simulink model "AT_and_specifications_artificial"  (R2019b)
settings: Solver=FixedStepAuto  StartTime=0.0  StopTime=10.0  FixedStep=fixedStepSize  RelTol=1e-3
settings Model: Creator=JEDDELAN  LastModifiedBy=jeddelan
settings DataIOCC: ReturnWorkspaceOutputs=off
settings DebuggingCC: ArithmeticOperatorsInVariantConditions=warning
settings SFSimCC: SimUseLocalCustomCode=off  CustomCodeUndefinedFunction=UseInterfaceOnly
settings RTWCC: RTWUseLocalCustomCode=off

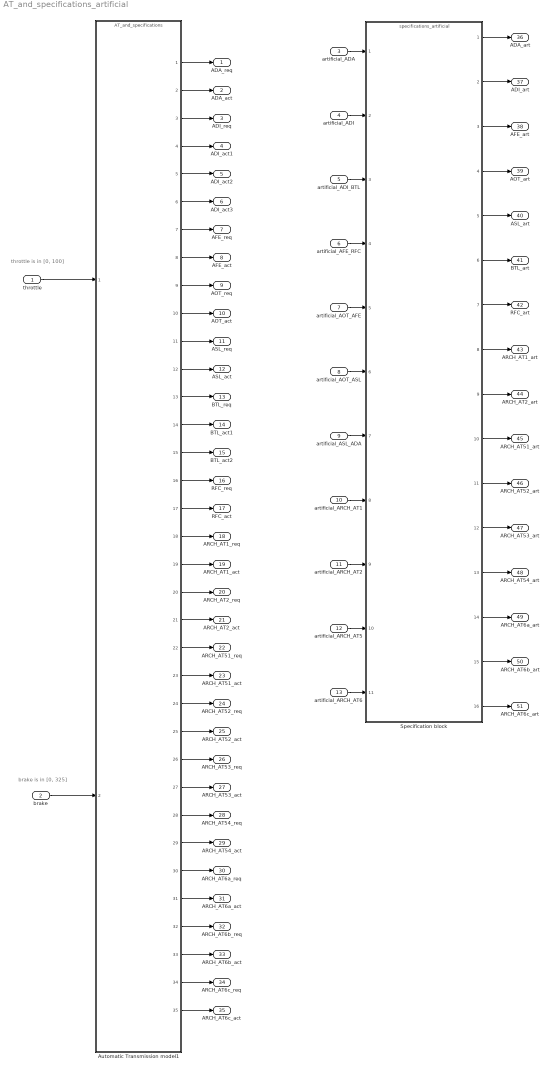
== system AT_and_specifications_artificial ==
  note: throttle is in [0, 100]
  note: brake is in [0, 325]
  throttle : Inport
  brake : Inport  Port=2
  artificial_ADA : Inport  Port=3
  artificial_ADI : Inport  Port=4
  artificial_ADI_BTL : Inport  Port=5
  artificial_AFE_RFC : Inport  Port=6
  artificial_AOT_AFE : Inport  Port=7
  artificial_AOT_ASL : Inport  Port=8
  artificial_ASL_ADA : Inport  Port=9
  artificial_ARCH_AT1 : Inport  Port=10
  artificial_ARCH_AT2 : Inport  Port=11
  artificial_ARCH_AT5 : Inport  Port=12
  artificial_ARCH_AT6 : Inport  Port=13
  Automatic Transmission model1 : ModelReference  ModelNameDialog=AT_and_specifications.slx  SimulationMode=Normal  ModelReferenceVersion=1.30
  Specification block : ModelReference  ModelNameDialog=specifications_artificial  SimulationMode=Normal  ModelReferenceVersion=1.52
  ADA_req : Outport  VectorParamsAs1DForOutWhenUnconnected=off
  ADA_act : Outport  Port=2  VectorParamsAs1DForOutWhenUnconnected=off
  ADI_req : Outport  Port=3  VectorParamsAs1DForOutWhenUnconnected=off
  ADI_act1 : Outport  Port=4  VectorParamsAs1DForOutWhenUnconnected=off
  ADI_act2 : Outport  Port=5  VectorParamsAs1DForOutWhenUnconnected=off
  ADI_act3 : Outport  Port=6  VectorParamsAs1DForOutWhenUnconnected=off
  AFE_req : Outport  Port=7  VectorParamsAs1DForOutWhenUnconnected=off
  AFE_act : Outport  Port=8  VectorParamsAs1DForOutWhenUnconnected=off
  AOT_req : Outport  Port=9  VectorParamsAs1DForOutWhenUnconnected=off
  AOT_act : Outport  Port=10  VectorParamsAs1DForOutWhenUnconnected=off
  ASL_req : Outport  Port=11  VectorParamsAs1DForOutWhenUnconnected=off
  ASL_act : Outport  Port=12  VectorParamsAs1DForOutWhenUnconnected=off
  BTL_req : Outport  Port=13  VectorParamsAs1DForOutWhenUnconnected=off
  BTL_act1 : Outport  Port=14  VectorParamsAs1DForOutWhenUnconnected=off
  BTL_act2 : Outport  Port=15  VectorParamsAs1DForOutWhenUnconnected=off
  RFC_req : Outport  Port=16  VectorParamsAs1DForOutWhenUnconnected=off
  RFC_act : Outport  Port=17  VectorParamsAs1DForOutWhenUnconnected=off
  ARCH_AT1_req : Outport  Port=18  VectorParamsAs1DForOutWhenUnconnected=off
  ARCH_AT1_act : Outport  Port=19  VectorParamsAs1DForOutWhenUnconnected=off
  ARCH_AT2_req : Outport  Port=20  VectorParamsAs1DForOutWhenUnconnected=off
  ARCH_AT2_act : Outport  Port=21  VectorParamsAs1DForOutWhenUnconnected=off
  ARCH_AT51_req : Outport  Port=22  VectorParamsAs1DForOutWhenUnconnected=off
  ARCH_AT51_act : Outport  Port=23  VectorParamsAs1DForOutWhenUnconnected=off
  ARCH_AT52_req : Outport  Port=24  VectorParamsAs1DForOutWhenUnconnected=off
  ARCH_AT52_act : Outport  Port=25  VectorParamsAs1DForOutWhenUnconnected=off
  ARCH_AT53_req : Outport  Port=26  VectorParamsAs1DForOutWhenUnconnected=off
  ARCH_AT53_act : Outport  Port=27  VectorParamsAs1DForOutWhenUnconnected=off
  ARCH_AT54_req : Outport  Port=28  VectorParamsAs1DForOutWhenUnconnected=off
  ARCH_AT54_act : Outport  Port=29  VectorParamsAs1DForOutWhenUnconnected=off
  ARCH_AT6a_req : Outport  Port=30  VectorParamsAs1DForOutWhenUnconnected=off
  ARCH_AT6a_act : Outport  Port=31  VectorParamsAs1DForOutWhenUnconnected=off
  ARCH_AT6b_req : Outport  Port=32  VectorParamsAs1DForOutWhenUnconnected=off
  ARCH_AT6b_act : Outport  Port=33  VectorParamsAs1DForOutWhenUnconnected=off
  ARCH_AT6c_req : Outport  Port=34  VectorParamsAs1DForOutWhenUnconnected=off
  ARCH_AT6c_act : Outport  Port=35  VectorParamsAs1DForOutWhenUnconnected=off
  ADA_art : Outport  Port=36  VectorParamsAs1DForOutWhenUnconnected=off
  ADI_art : Outport  Port=37  VectorParamsAs1DForOutWhenUnconnected=off
  AFE_art : Outport  Port=38  VectorParamsAs1DForOutWhenUnconnected=off
  AOT_art : Outport  Port=39  VectorParamsAs1DForOutWhenUnconnected=off
  ASL_art : Outport  Port=40  VectorParamsAs1DForOutWhenUnconnected=off
  BTL_art : Outport  Port=41  VectorParamsAs1DForOutWhenUnconnected=off
  RFC_art : Outport  Port=42  VectorParamsAs1DForOutWhenUnconnected=off
  ARCH_AT1_art : Outport  Port=43  VectorParamsAs1DForOutWhenUnconnected=off
  ARCH_AT2_art : Outport  Port=44  VectorParamsAs1DForOutWhenUnconnected=off
  ARCH_AT51_art : Outport  Port=45  VectorParamsAs1DForOutWhenUnconnected=off
  ARCH_AT52_art : Outport  Port=46  VectorParamsAs1DForOutWhenUnconnected=off
  ARCH_AT53_art : Outport  Port=47  VectorParamsAs1DForOutWhenUnconnected=off
  ARCH_AT54_art : Outport  Port=48  VectorParamsAs1DForOutWhenUnconnected=off
  ARCH_AT6a_art : Outport  Port=49  VectorParamsAs1DForOutWhenUnconnected=off
  ARCH_AT6b_art : Outport  Port=50  VectorParamsAs1DForOutWhenUnconnected=off
  ARCH_AT6c_art : Outport  Port=51  VectorParamsAs1DForOutWhenUnconnected=off
  wires:
  throttle/1 -> Automatic Transmission model1/1
  brake/1 -> Automatic Transmission model1/2
  Automatic Transmission model1/17 -> RFC_act/1
  Automatic Transmission model1/18 -> ARCH_AT1_req/1
  Automatic Transmission model1/19 -> ARCH_AT1_act/1
  Automatic Transmission model1/20 -> ARCH_AT2_req/1
  Automatic Transmission model1/21 -> ARCH_AT2_act/1
  Automatic Transmission model1/35 -> ARCH_AT6c_act/1
  Automatic Transmission model1/34 -> ARCH_AT6c_req/1
  Automatic Transmission model1/33 -> ARCH_AT6b_act/1
  Automatic Transmission model1/32 -> ARCH_AT6b_req/1
  Automatic Transmission model1/31 -> ARCH_AT6a_act/1
  Automatic Transmission model1/30 -> ARCH_AT6a_req/1
  Automatic Transmission model1/29 -> ARCH_AT54_act/1
  Automatic Transmission model1/28 -> ARCH_AT54_req/1
  Automatic Transmission model1/27 -> ARCH_AT53_act/1
  Specification block/3 -> AFE_art/1
  Specification block/2 -> ADI_art/1
  Specification block/1 -> ADA_art/1
  Specification block/4 -> AOT_art/1
  Specification block/5 -> ASL_art/1
  Specification block/6 -> BTL_art/1
  Specification block/7 -> RFC_art/1
  Specification block/8 -> ARCH_AT1_art/1
  Specification block/9 -> ARCH_AT2_art/1
  Specification block/10 -> ARCH_AT51_art/1
  Specification block/11 -> ARCH_AT52_art/1
  Specification block/12 -> ARCH_AT53_art/1
  Specification block/13 -> ARCH_AT54_art/1
  Specification block/14 -> ARCH_AT6a_art/1
  Specification block/15 -> ARCH_AT6b_art/1
  Specification block/16 -> ARCH_AT6c_art/1
  Automatic Transmission model1/26 -> ARCH_AT53_req/1
  Automatic Transmission model1/25 -> ARCH_AT52_act/1
  Automatic Transmission model1/24 -> ARCH_AT52_req/1
  Automatic Transmission model1/23 -> ARCH_AT51_act/1
  Automatic Transmission model1/22 -> ARCH_AT51_req/1
  Automatic Transmission model1/16 -> RFC_req/1
  Automatic Transmission model1/15 -> BTL_act2/1
  Automatic Transmission model1/14 -> BTL_act1/1
  Automatic Transmission model1/13 -> BTL_req/1
  Automatic Transmission model1/12 -> ASL_act/1
  Automatic Transmission model1/11 -> ASL_req/1
  Automatic Transmission model1/10 -> AOT_act/1
  Automatic Transmission model1/9 -> AOT_req/1
  Automatic Transmission model1/8 -> AFE_act/1
  Automatic Transmission model1/7 -> AFE_req/1
  Automatic Transmission model1/6 -> ADI_act3/1
  Automatic Transmission model1/5 -> ADI_act2/1
  Automatic Transmission model1/4 -> ADI_act1/1
  Automatic Transmission model1/3 -> ADI_req/1
  Automatic Transmission model1/2 -> ADA_act/1
  Automatic Transmission model1/1 -> ADA_req/1
  artificial_ADA/1 -> Specification block/1
  artificial_ADI/1 -> Specification block/2
  artificial_ADI_BTL/1 -> Specification block/3
  artificial_AFE_RFC/1 -> Specification block/4
  artificial_AOT_AFE/1 -> Specification block/5
  artificial_AOT_ASL/1 -> Specification block/6
  artificial_ASL_ADA/1 -> Specification block/7
  artificial_ARCH_AT1/1 -> Specification block/8
  artificial_ARCH_AT2/1 -> Specification block/9
  artificial_ARCH_AT5/1 -> Specification block/10
  artificial_ARCH_AT6/1 -> Specification block/11
